simulink model "twolinkenv"  (R2019a)
settings: Solver=VariableStepAuto  StartTime=0.0  StopTime=25  RelTol=1e-3
model workspace (MATLAB code in the model file):
  | mCart = 1;
  | mPend = 1;
  | g = 9.81;
  | L = 0.5;
  | theta0 = 180;
  | Kd = 10;
undefined symbols (not defined in the file or in its folder): epinum
libraries: aerolibconvert2 x3, rllib x1
settings Model: OrderedModelArguments=off  Creator=ndoshi  LastModifiedBy=hoomaan
settings DataIOCC: TimeSaveName=T  SignalLoggingName=LoggedSigs
settings DebuggingCC: ArithmeticOperatorsInVariantConditions=warning

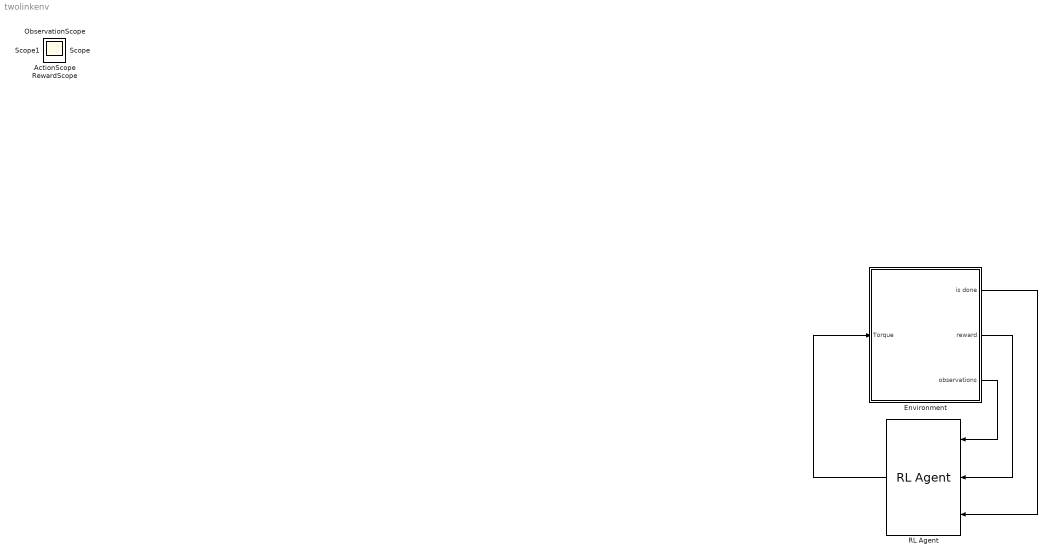
== system twolinkenv ==
  Environment : Subsystem
  RL Agent : rllib/RL Agent  Agent=agent  ProvideReward=on  ProvideIsDone=on  ProvideCumRwd=off  TreatAsDirectFeedthrough=on  CollectLoggedSignals=on  CollectModelStates=on
      settings: SourceProductName=Reinforcement Learning Toolbox
  ActionScope : Scope
  ObservationScope : Scope
  RewardScope : Scope
  Scope : Scope
  Scope1 : Scope
  wires:
  RL Agent/1 -> Environment/1(Torque)
  Environment/3(observations) -> RL Agent/1
  Environment/2(reward) -> RL Agent/2
  Environment/1(is done) -> RL Agent/3

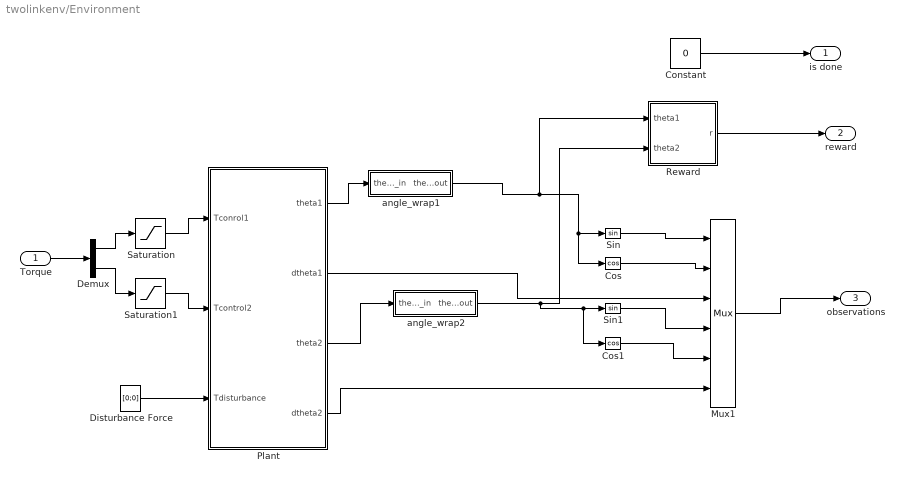
== system twolinkenv/Environment ==
  Torque : Inport
  Constant : Constant  Value=0
  Cos : Trigonometry  Operator=cos
  Cos1 : Trigonometry  Operator=cos
  Demux : Demux  Outputs=2
  Disturbance Force : Constant  Value=[0;0]
  Mux1 : Mux  Inputs=6
  Plant : Subsystem
  Reward : Subsystem
  Saturation : Saturate  UpperLimit=15  LowerLimit=-15
  Saturation1 : Saturate  UpperLimit=15  LowerLimit=-15
  Sin : Trigonometry
  Sin1 : Trigonometry
  angle_wrap1 : Subsystem
  angle_wrap2 : Subsystem
  is done : Outport
  reward : Outport  Port=2
  observations : Outport  Port=3
  wires:
  Mux1/1 -> observations/1
  Plant/1(theta1) -> angle_wrap1/1(theta_in)
  Disturbance Force/1 -> Plant/3(Tdisturbance)
  Sin/1 -> Mux1/1
  Cos/1 -> Mux1/2
  Reward/1(r) -> reward/1
  Saturation/1 -> Plant/1(Tconrol1)
  angle_wrap1/1(theta_out) -> Reward/1(theta1), Cos/1, Sin/1
  Plant/3(theta2) -> angle_wrap2/1(theta_in)
  angle_wrap2/1(theta_out) -> Reward/2(theta2), Cos1/1, Sin1/1
  Sin1/1 -> Mux1/4
  Cos1/1 -> Mux1/5
  Plant/4(dtheta2) -> Mux1/6
  Plant/2(dtheta1) -> Mux1/3
  Constant/1 -> is done/1
  Saturation1/1 -> Plant/2(Tcontrol2)
  Torque/1 -> Demux/1
  Demux/1 -> Saturation/1
  Demux/2 -> Saturation1/1

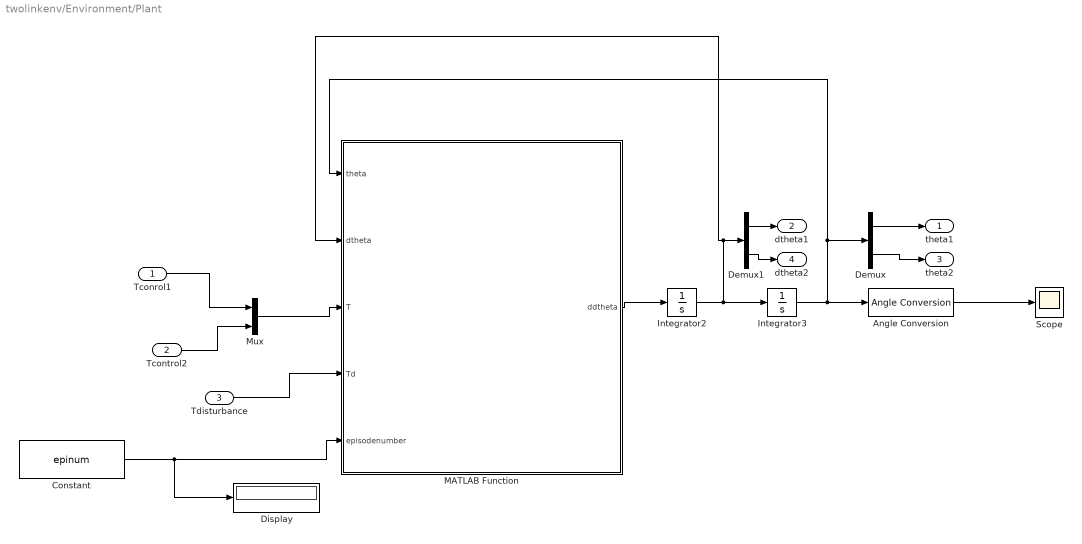
== system twolinkenv/Environment/Plant ==
  Tconrol1 : Inport
  Tcontrol2 : Inport  Port=2
  Tdisturbance : Inport  Port=3
  Angle Conversion : aerolibconvert2/Angle Conversion  IU=rad  OU=deg
  Constant : Constant  Value=epinum
  Demux : Demux  Outputs=2
  Demux1 : Demux  Outputs=2
  Display : Display
  Integrator2 : Integrator  InitialCondition=zeros(2,1)
  Integrator3 : Integrator  InitialCondition=[-pi/2;0]
  MATLAB Function : MATLAB Function  TreatAsAtomicUnit=on
  Mux : Mux  Inputs=2
  Scope : Scope
  theta1 : Outport
  dtheta1 : Outport  Port=2
  theta2 : Outport  Port=3
  dtheta2 : Outport  Port=4
  wires:
  Integrator2/1 -> Integrator3/1, Demux1/1, MATLAB Function/2(dtheta)
  MATLAB Function/1(ddtheta) -> Integrator2/1
  Integrator3/1 -> MATLAB Function/1(theta), Demux/1, Angle Conversion/1
  Angle Conversion/1 -> Scope/1
  Demux1/1 -> dtheta1/1
  Demux/1 -> theta1/1
  Demux1/2 -> dtheta2/1
  Demux/2 -> theta2/1
  Tconrol1/1 -> Mux/1
  Mux/1 -> MATLAB Function/3(T)
  Tcontrol2/1 -> Mux/2
  Tdisturbance/1 -> MATLAB Function/4(Td)
  Constant/1 -> MATLAB Function/5(episodenumber), Display/1

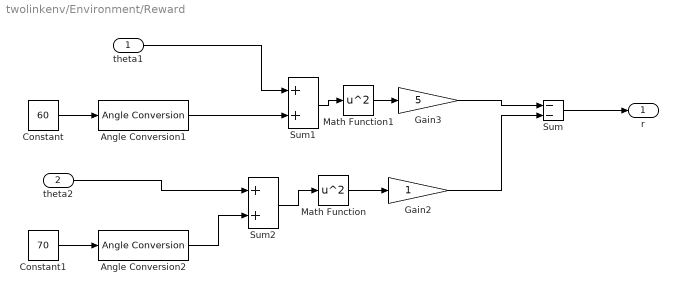
== system twolinkenv/Environment/Reward ==
  theta1 : Inport
  theta2 : Inport  Port=2
  Angle Conversion1 : aerolibconvert2/Angle Conversion  IU=deg  OU=rad
  Angle Conversion2 : aerolibconvert2/Angle Conversion  IU=deg  OU=rad
  Constant : Constant  Value=60
  Constant1 : Constant  Value=70
  Gain2 : Gain
  Gain3 : Gain  Gain=5
  Math Function : Math  Operator=square  SaturateOnIntegerOverflow=on
  Math Function1 : Math  Operator=square  SaturateOnIntegerOverflow=on
  Sum : Sum  Inputs=--
  Sum1 : Sum
  Sum2 : Sum
  r : Outport
  wires:
  Gain2/1 -> Sum/2
  Math Function/1 -> Gain2/1
  Sum/1 -> r/1
  Sum1/1 -> Math Function1/1
  Constant/1 -> Angle Conversion1/1
  Angle Conversion1/1 -> Sum1/2
  Math Function1/1 -> Gain3/1
  Gain3/1 -> Sum/1
  Sum2/1 -> Math Function/1
  Constant1/1 -> Angle Conversion2/1
  Angle Conversion2/1 -> Sum2/2
  theta1/1 -> Sum1/1
  theta2/1 -> Sum2/1

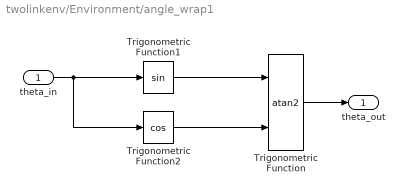
== system twolinkenv/Environment/angle_wrap1 ==
  theta_in : Inport
  Trigonometric Function : Trigonometry  Operator=atan2
  Trigonometric Function1 : Trigonometry
  Trigonometric Function2 : Trigonometry  Operator=cos
  theta_out : Outport
  wires:
  Trigonometric Function2/1 -> Trigonometric Function/2
  Trigonometric Function1/1 -> Trigonometric Function/1
  Trigonometric Function/1 -> theta_out/1
  theta_in/1 -> Trigonometric Function1/1, Trigonometric Function2/1

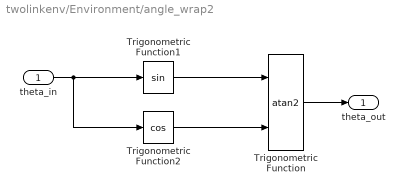
== system twolinkenv/Environment/angle_wrap2 ==
  theta_in : Inport
  Trigonometric Function : Trigonometry  Operator=atan2
  Trigonometric Function1 : Trigonometry
  Trigonometric Function2 : Trigonometry  Operator=cos
  theta_out : Outport
  wires:
  theta_in/1 -> Trigonometric Function2/1, Trigonometric Function1/1
  Trigonometric Function/1 -> theta_out/1
  Trigonometric Function1/1 -> Trigonometric Function/1
  Trigonometric Function2/1 -> Trigonometric Function/2

== matlab function twolinkenv/Environment/Plant/MATLAB Function ==
  data: theta input; ddtheta output; dtheta input; T input; Td input; episodenumber input
function ddtheta  = fcn(theta,dtheta,T,Td,episodenumber)
theta1=theta(1);theta2=theta(2);
dtheta1=dtheta(1);dtheta2=dtheta(2);
m1=3.9775;
% m22=2.84;
l1=0.432;
% l22=0.432;
g=9.81;
c1=10.8;
c2=3.2;

if episodenumber<20
    m22=2.84;
    l22=0.432;
else
    m22=2.84/2;
    l22=0.432/2;
end

a=l22^2*m22+l1^2*(m1+m22);
b=2*l1*l22*m22;
c=l22^2*m22;
d=(m1+m22)*l1*g;
e=m22*l22*g;


M=[a+b*cos(theta2) c+b*cos(theta2)/2;...
    c+b*cos(theta2)/2 c];
V=[-b*dtheta2*sin(theta2) -b*dtheta2*sin(theta2)/2;...
    b*dtheta1*sin(theta2)/2 0];
G=[d*cos(theta1)+e*cos(theta1+theta2);e*cos(theta1+theta2)];
F=[c1*dtheta1;c2*dtheta2];
ddtheta=inv(M)*(-V*dtheta-G-F-Td+T);
